simulink model "LQR"  (R2017b)
settings: Solver=VariableStepAuto  StartTime=0.0  StopTime=10.0  RelTol=1e-3
values from neighbouring files (symbols this model uses):
  K = [-31.6227766017 -36.1124465891 1641.52806915 127.188184677]    [matlab.mat]
settings Model: Creator=DELL  LastModifiedBy=DELL

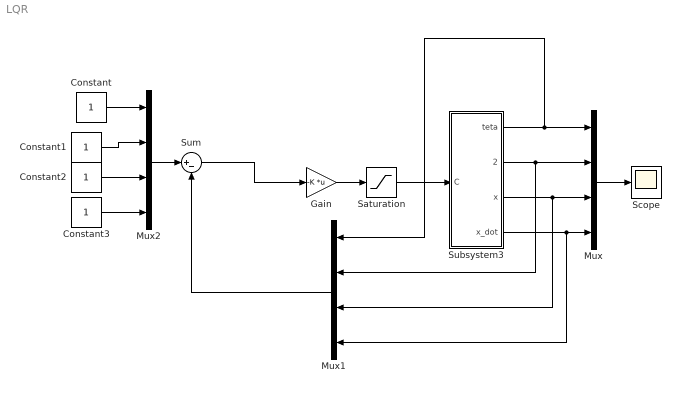
== system LQR ==
  Constant{,1..3} (4 alike) : Constant
  Gain : Gain  Gain=-K  Multiplication=Matrix(K*u)
  Mux : Mux
  Mux1 : Mux
  Mux2 : Mux
  Saturation : Saturate
  Scope : Scope
  Subsystem3 : Subsystem
  Sum : Sum  Inputs=|+-
  wires:
  Subsystem3/1(teta) -> Mux1/1, Mux/1
  Subsystem3/2(teta_dot) -> Mux1/2, Mux/2
  Subsystem3/3(x) -> Mux1/3, Mux/3
  Subsystem3/4(x_dot) -> Mux1/4, Mux/4
  Mux/1 -> Scope/1
  Saturation/1 -> Subsystem3/1(C)
  Gain/1 -> Saturation/1
  Mux1/1 -> Sum/2
  Mux2/1 -> Sum/1
  Constant3/1 -> Mux2/4
  Constant2/1 -> Mux2/3
  Constant/1 -> Mux2/1
  Constant1/1 -> Mux2/2
  Sum/1 -> Gain/1

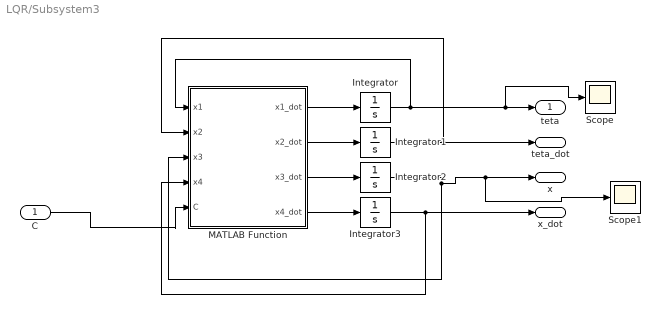
== system LQR/Subsystem3 ==
  C : Inport
  Integrator : Integrator  InitialCondition=0.014
  Integrator1 : Integrator
  Integrator2 : Integrator  InitialCondition=0.03
  Integrator3 : Integrator
  MATLAB Function : MATLAB Function  TreatAsAtomicUnit=on
  Scope : Scope
  Scope1 : Scope
  teta : Outport
  teta_dot : Outport  Port=2
  x : Outport  Port=3
  x_dot : Outport  Port=4
  wires:
  MATLAB Function/2(x2_dot) -> Integrator1/1
  Integrator/1 -> teta/1, Scope/1, MATLAB Function/1(x1)
  MATLAB Function/4(x4_dot) -> Integrator3/1
  MATLAB Function/3(x3_dot) -> Integrator2/1
  MATLAB Function/1(x1_dot) -> Integrator/1
  Integrator1/1 -> teta_dot/1, MATLAB Function/2(x2)
  Integrator2/1 -> x/1, Scope1/1, MATLAB Function/3(x3)
  Integrator3/1 -> x_dot/1, MATLAB Function/4(x4)
  C/1 -> MATLAB Function/5(C)

== matlab function LQR/Subsystem3/MATLAB Function ==
  data: x1 input; x1_dot output; x2 input; x3 input; x4 input; C input; x2_dot output; x3_dot output; x4_dot output
function [x1_dot,x2_dot,x3_dot,x4_dot] = fcn(x1,x2,x3,x4,C)
Mw=0.5;
Mb=7;
R=0.07;
L=0.3;
D=0.41;
g=9.8;
x1_dot=x2;
x2_dot=(-0.75*g*sin(x1)/L)/((0.75*(Mw*R+Mb*L*cos(x1))*cos(x1)/((2*Mw+Mb)*L))-1)+...
    (0.75*Mb*L*sin(x1)*cos(x1)*(x2^2)/(L*(2*Mw+Mb)))/((0.75*(Mw*R+Mb*L*cos(x1))*cos(x1)/((2*Mw+Mb)*L))-1)+...
 C*(0.75*(Mw*R+Mb*L*cos(x1))*(1+(sin(x1)^2))/(Mb*L^2)+1/R)/(2*Mw+Mb-(0.75*(Mw*R+Mb*L*cos(x1))*cos(x1)/L));


x3_dot=x4;
x4_dot=(-0.75*g*(Mw*R+Mb*L*cos(x1))*sin(x1)/L)/(2*Mw+Mb-(0.75*(Mw*R+Mb*L*cos(x1))*cos(x1)/L))+...
    (Mb*L*sin(x1)*(x2^2))/((2*Mw+Mb-(0.75*(Mw*R+Mb*L*cos(x1))*cos(x1)/L)))+...
    C*((0.75*(Mw*R+Mb*L*cos(x1))*(1+(sin(x1)^2))/(Mb*L))+(1/R))/((2*Mw+Mb-(0.75*(Mw*R+Mb*L*cos(x1))*cos(x1)/L)));
